simulink model "counter_ref"  (Simulink 4.00)
settings: Solver=FixedStepDiscrete  StartTime=0.0  StopTime=30  RelTol=1e-3
PostLoadFcn:
  | set_param(gcs,'SimulationCommand','Update')
undefined symbols (not defined in the file or in its folder): High
libraries: dspswit3 x2
settings Model: RequirementInfo=9  Creator=ckamachi  LastModifiedBy=ckamachi  SaveTime=off  LimitDataPoints=off  ExtModeTrigMode=oneshot  ExtModeArmWhenConnect=off  BlockReductionOpt=off

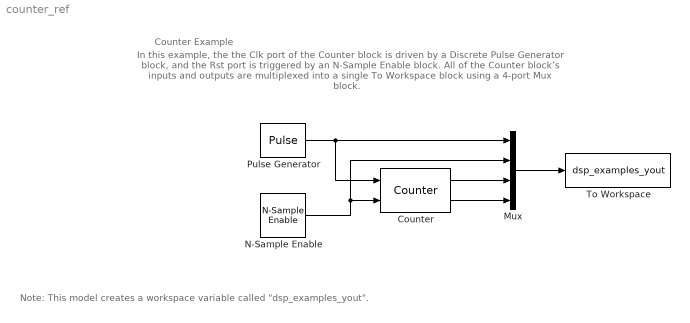
== system counter_ref ==
  note: Counter Example
  note: In this example, the the Clk port of the Counter block is driven by a
      | Discrete Pulse Generator block, and the Rst port is triggered by an
      | N-Sample Enable block. All of the Counter block’s inputs and outputs
      | are multiplexed into a single To Workspace block using a 4-port Mux block.
  note: Note: This model creates a workspace variable called "dsp_examples_yout".
  Counter : dspswit3/Counter  Direction=Down  CountEvent=Rising edge  CounterSize=User defined  MaxCount=20  InitialCount=5  Output=Count and Hit  HitValue=4  ResetInput=on  SamplesPerFrame=1  Ts=1
  Mux : Mux  Inputs=4
  N-Sample Enable : dspswit3/N-Sample Enable  N=6  ActiveLevel=High (1)  reset=off  TriggerType=Rising edge  Ts=1
  Pulse Generator : DiscretePulseGenerator  PulseType=Sample-based  Amplitude=1  Period=2  PulseWidth=1  PhaseDelay=0  SampleTime=1
  To Workspace : ToWorkspace  VariableName=dsp_examples_yout  SampleTime=-1  SaveFormat=Array
  wires:
  Counter/2 -> Mux/4
  Counter/1 -> Mux/3
  Pulse Generator/1 -> Mux/1, Counter/1
  N-Sample Enable/1 -> Counter/2, Mux/2
  Mux/1 -> To Workspace/1
